simulink model "clutch_trial"  (R2024b)
settings: Solver=ode1be  StartTime=0.0  StopTime=4  FixedStep=0.01  RelTol=1e-3
undefined symbols (not defined in the file or in its folder): J_load, J_rotor, mi_c, mi_s, N_clutch, r_eq_clutch, rpm_in, sigma0, sigma1, sigma2, time, vs
libraries: simulink x3
settings Model: Creator=menda  LastModifiedBy=menda

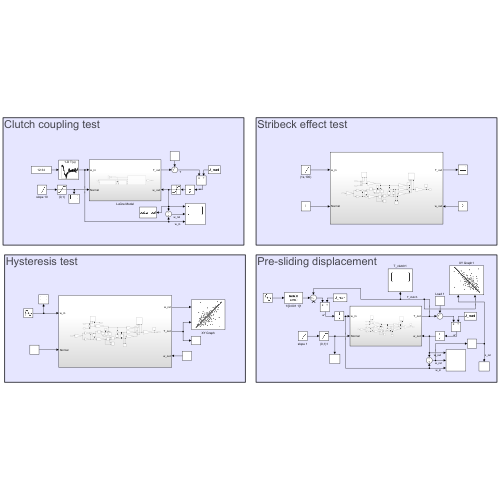
[thumbnail: Simulink's stored preview of the top-level diagram]
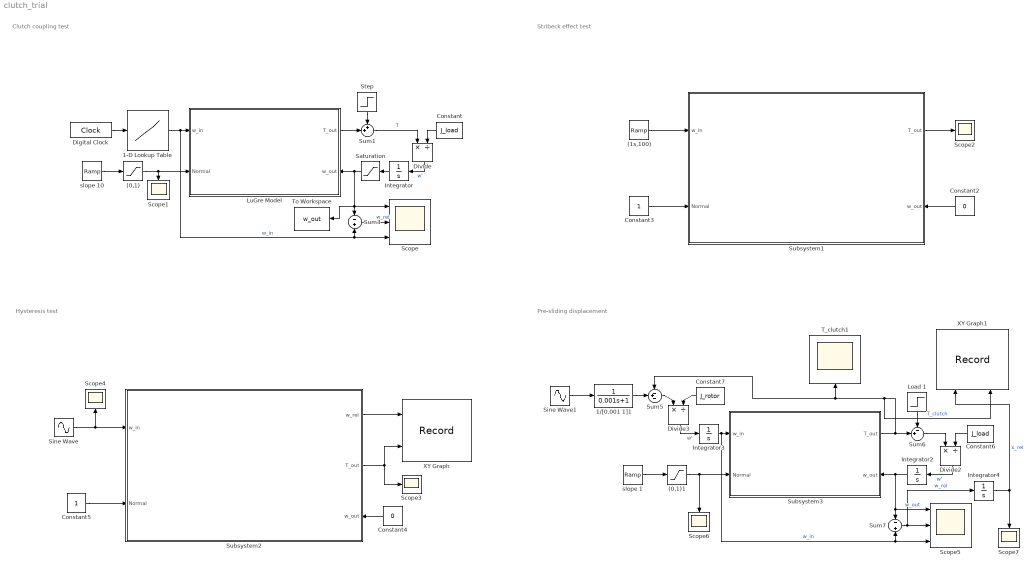
== system clutch_trial ==
  note: Clutch coupling test
  note: Stribeck effect test
  note: Hysteresis test
  note: Pre-sliding displacement
  (0,1) : Saturate  UpperLimit=1  LowerLimit=0
  (0,1)1 : Saturate  UpperLimit=1  LowerLimit=0
  (1s,100) : simulink/Sources/Ramp  slope=100  start=1  InitialOutput=0
  1-D Lookup Table : Lookup_n-D  NumberOfTableDimensions=1  BreakpointsForDimension1=time  Table=rpm_in  InternalRulePriority=Speed  RndMeth=Simplest
  1/[0.001 1]1 : TransferFcn  Denominator=[0.001 1]
  Constant : Constant  Value=J_load
  Constant2 : Constant  Value=0
  Constant3 : Constant
  Constant4 : Constant  Value=0
  Constant5 : Constant
  Constant6 : Constant  Value=J_load
  Constant7 : Constant  Value=J_rotor
  Digital Clock : DigitalClock  SampleTime=0.01
  Divide : Product  Inputs=*/
  Divide2 : Product  Inputs=*/
  Divide3 : Product  Inputs=*/
  Integrator{,2..4} (4 alike) : Integrator
  Load 1 : Step  Time=0  After=0  SampleTime=0
  LuGre Model : Subsystem
      settings: PortSchema="{\"entries\":[{\"content\":{\"sides\":[{\"content\":{\"connectorIds\":[\"In1\",\"In2\"]},\"type\":\"ConnectorPlacement.EquallySpacedRectSide\",\"uuid\":\"4a43e1ea-51cc-4f14-abc2-c6b93b5ec80a\"},{\"content\":{\"connectorIds\":[\"Out1\",\"In3\"],\"side\":\"RIGHT\"},\"type\":\"ConnectorPlacement.EquallySpacedRectSide\",\"uuid\":\"02b73943-aa72-4ec9-9088-698ba8727517\"},{\"content\":{\"side\":\"TOP\"},\"type\":\"ConnectorPlacement.EquallySpacedRectSide\",\"uuid\":\"deeff554-d171-484d-b470-fd1118263e94\"}]},\"type\":\"ConnectorPlacement.EquallySpacedConnector\",\"uuid\":\"dd3f8be3-8b87-48df-afb6-ff993e210eb5\"}],\"packageUris\":[\"http://schema.mathworks.com/mf0/Connector/R2020b\"],\"version\":\"1.0\"}"
  Saturation : Saturate  UpperLimit=inf  LowerLimit=0
  Scope : Scope  NumInputPorts=3
  Scope{1..4,6..7} (6 alike) : Scope
  Scope5 : Scope  NumInputPorts=3
  Sine Wave : Sin  Amplitude=30  Frequency=2  SampleTime=0
  Sine Wave1 : Sin  Amplitude=5  SampleTime=0
  Step : Step  Time=0  After=-10  SampleTime=0
  Subsystem1 : Subsystem
      settings: PortSchema="{\"entries\":[{\"content\":{\"sides\":[{\"content\":{\"connectorIds\":[\"In1\",\"In2\"]},\"type\":\"ConnectorPlacement.EquallySpacedRectSide\",\"uuid\":\"4a43e1ea-51cc-4f14-abc2-c6b93b5ec80a\"},{\"content\":{\"connectorIds\":[\"Out1\",\"In3\"],\"side\":\"RIGHT\"},\"type\":\"ConnectorPlacement.EquallySpacedRectSide\",\"uuid\":\"02b73943-aa72-4ec9-9088-698ba8727517\"},{\"content\":{\"side\":\"TOP\"},\"type\":\"ConnectorPlacement.EquallySpacedRectSide\",\"uuid\":\"deeff554-d171-484d-b470-fd1118263e94\"}]},\"type\":\"ConnectorPlacement.EquallySpacedConnector\",\"uuid\":\"dd3f8be3-8b87-48df-afb6-ff993e210eb5\"}],\"packageUris\":[\"http://schema.mathworks.com/mf0/Connector/R2020b\"],\"version\":\"1.0\"}"
  Subsystem2 : Subsystem
      settings: PortSchema="{\"entries\":[{\"content\":{\"sides\":[{\"content\":{\"connectorIds\":[\"In1\",\"In2\"]},\"type\":\"ConnectorPlacement.EquallySpacedRectSide\",\"uuid\":\"4a43e1ea-51cc-4f14-abc2-c6b93b5ec80a\"},{\"content\":{\"connectorIds\":[\"Out1\",\"Out2\",\"In3\"],\"side\":\"RIGHT\"},\"type\":\"ConnectorPlacement.EquallySpacedRectSide\",\"uuid\":\"02b73943-aa72-4ec9-9088-698ba8727517\"},{\"content\":{\"side\":\"TOP\"},\"type\":\"ConnectorPlacement.EquallySpacedRectSide\",\"uuid\":\"deeff554-d171-484d-b470-fd1118263e94\"}]},\"type\":\"ConnectorPlacement.EquallySpacedConnector\",\"uuid\":\"dd3f8be3-8b87-48df-afb6-ff993e210eb5\"}],\"packageUris\":[\"http://schema.mathworks.com/mf0/Connector/R2020b\"],\"version\":\"1.0\"}"
  Subsystem3 : Subsystem
      settings: PortSchema="{\"entries\":[{\"content\":{\"sides\":[{\"content\":{\"connectorIds\":[\"In1\",\"In2\"]},\"type\":\"ConnectorPlacement.EquallySpacedRectSide\",\"uuid\":\"4a43e1ea-51cc-4f14-abc2-c6b93b5ec80a\"},{\"content\":{\"connectorIds\":[\"Out1\",\"In3\"],\"side\":\"RIGHT\"},\"type\":\"ConnectorPlacement.EquallySpacedRectSide\",\"uuid\":\"02b73943-aa72-4ec9-9088-698ba8727517\"},{\"content\":{\"side\":\"TOP\"},\"type\":\"ConnectorPlacement.EquallySpacedRectSide\",\"uuid\":\"deeff554-d171-484d-b470-fd1118263e94\"}]},\"type\":\"ConnectorPlacement.EquallySpacedConnector\",\"uuid\":\"dd3f8be3-8b87-48df-afb6-ff993e210eb5\"}],\"packageUris\":[\"http://schema.mathworks.com/mf0/Connector/R2020b\"],\"version\":\"1.0\"}"
  Sum1 : Sum  Inputs=++|
  Sum3 : Sum  Inputs=-|+
  Sum5 : Sum  Inputs=-+-
  Sum6 : Sum  Inputs=-+|
  Sum7 : Sum  Inputs=-|+
  T_clutch1 : Scope
  To Workspace : ToWorkspace  VariableName=w_out  SampleTime=-1
  XY Graph : Record  FileSettingsInternal="{\"entries\":[{\"content\":{\"excelSettings\":{\"content\":{},\"type\":\"Streamout.ExcelSettings\"}},\"type\":\"Streamout.FileSettingStorage\",\"uuid\":\"\"}],\"packageUris\":[\"http:\\/\\/schema.mathworks.com\\/mf0\\/streamout_blocks\\/R2020a\"],\"version\":\"1.0\"}"  Layout=[1 1]  SignalsInternal="{\"entries\":[{\"content\":{\"signals\":[{\"content\":{\"blockPath\":[],\"dimensions\":[1],\"domain\":\"\",\"lineColor\":\"#a2142f\",\"plots\":[ 1 ],\"port\":1,\"sid\":[\"\"],\"signalID\":1,\"signalName\":\"Subsystem2:1\"},\"type\":\"RecordBlkView.Signal\",\"uuid\":\"\"},{\"content\":{\"blockPath\":[],\"dimensions\":[1],\"domain\":\"\",\"lineColor\":\"#139fff\",\"plots\":[ 1 ],\"port\":2,\"sid\":[\"\"],\"signalID\":2,\"signalName\":\"Subsystem2:2\"},\"type\":\"RecordBlkView.Signal\",\"uuid\":\"\"}]},\"type\":\"RecordBlkView.InputSignals\",\"uuid\":\"\"}],\"packageUris\":[\"http:\\/\\/schema.mathworks.com\\/mf0\\/streamout_blocks\\/R2020a\"],\"version\":\"1.0\"}"  VisualizationBindings="{\"xyplotplugin\":{\"info\":[{\"series\":[{\"bindingParametersList\":[{\"parameter\":\"X-Axis\",\"signalID\":1,\"signalName\":\"Subsystem2:1\"},{\"parameter\":\"Y-Axis\",\"signalID\":2,\"signalName\":\"Subsystem2:2\"}],\"seriesID\":0}],\"subplotID\":1}]}}"  CompatibilityTag=XY
  XY Graph1 : Record  FileSettingsInternal="{\"entries\":[{\"content\":{\"excelSettings\":{\"content\":{},\"type\":\"Streamout.ExcelSettings\"}},\"type\":\"Streamout.FileSettingStorage\",\"uuid\":\"\"}],\"packageUris\":[\"http:\\/\\/schema.mathworks.com\\/mf0\\/streamout_blocks\\/R2020a\"],\"version\":\"1.0\"}"  Layout=[1 1]  SignalsInternal="{\"entries\":[{\"content\":{\"signals\":[{\"content\":{\"blockPath\":[],\"dimensions\":[1],\"domain\":\"\",\"lineColor\":\"#a2142f\",\"plots\":[ 1 ],\"port\":1,\"sid\":[\"\"],\"signalID\":1,\"signalName\":\"x_rel\"},\"type\":\"RecordBlkView.Signal\",\"uuid\":\"\"},{\"content\":{\"blockPath\":[],\"dimensions\":[1],\"domain\":\"\",\"lineColor\":\"#139fff\",\"plots\":[ 1 ],\"port\":2,\"sid\":[\"\"],\"signalID\":2,\"signalName\":\"T_clutch\"},\"type\":\"RecordBlkView.Signal\",\"uuid\":\"\"}]},\"type\":\"RecordBlkView.InputSignals\",\"uuid\":\"\"}],\"packageUris\":[\"http:\\/\\/schema.mathworks.com\\/mf0\\/streamout_blocks\\/R2020a\"],\"version\":\"1.0\"}"  VisualizationBindings="{\"xyplotplugin\":{\"info\":[{\"series\":[{\"bindingParametersList\":[{\"parameter\":\"X-Axis\",\"signalID\":1,\"signalName\":\"x_rel\"},{\"parameter\":\"Y-Axis\",\"signalID\":2,\"signalName\":\"T_clutch\"}],\"seriesID\":0}],\"subplotID\":1}]}}"  CompatibilityTag=XY
  slope 1 : simulink/Sources/Ramp  slope=10  start=0  InitialOutput=0
  slope 10 : simulink/Sources/Ramp  slope=1  start=0.7  InitialOutput=0
  wires:
  1-D Lookup Table/1 -> Scope/3, Sum3/2, LuGre Model/1(w_in)  "w_in"
  Integrator/1 -> Saturation/1
  Divide/1 -> Integrator/1  "w'"
  slope 10/1 -> (0,1)/1
  (0,1)/1 -> LuGre Model/2(Normal), Scope1/1
  Subsystem1/1(T_out) -> Scope2/1
  Constant2/1 -> Subsystem1/3(w_out)
  Constant3/1 -> Subsystem1/2(Normal)
  (1s,100)/1 -> Subsystem1/1(w_in)
  LuGre Model/1(T_out) -> Sum1/2
  Constant/1 -> Divide/2
  Constant5/1 -> Subsystem2/2(Normal)
  Constant4/1 -> Subsystem2/3(w_out)
  Subsystem2/2(T_out) -> XY Graph/2, Scope3/1
  Sine Wave/1 -> Subsystem2/1(w_in), Scope4/1
  Sum3/1 -> Scope/2  "w_rel"
  Subsystem2/1(w_rel) -> XY Graph/1
  Sum7/1 -> Integrator4/1, Scope5/2  "w_rel"
  Constant6/1 -> Divide2/2
  Sum6/1 -> Divide2/1
  Load 1/1 -> Sum6/1
  1/[0.001 1]1/1 -> Sum5/2
  Sum5/1 -> Divide3/1
  Constant7/1 -> Divide3/2
  Sine Wave1/1 -> 1/[0.001 1]1/1
  (0,1)1/1 -> Scope6/1, Subsystem3/2(Normal)
  Divide3/1 -> Integrator3/1  "w'"
  slope 1/1 -> (0,1)1/1
  Divide2/1 -> Integrator2/1  "w'"
  Subsystem3/1(T_out) -> Sum6/2, T_clutch1/1, Sum5/1, XY Graph1/2  "T_clutch"
  Integrator2/1 -> Scope5/1, Sum7/1, Subsystem3/3(w_out)  "w_out"
  Integrator3/1 -> Subsystem3/1(w_in), Sum7/2, Scope5/3  "w_in"
  Integrator4/1 -> Scope7/1, XY Graph1/1  "x_rel"
  Digital Clock/1 -> 1-D Lookup Table/1
  Sum1/1 -> Divide/1  "T"
  Step/1 -> Sum1/1
  Saturation/1 -> To Workspace/1, Sum3/1, Scope/1, LuGre Model/3(w_out)

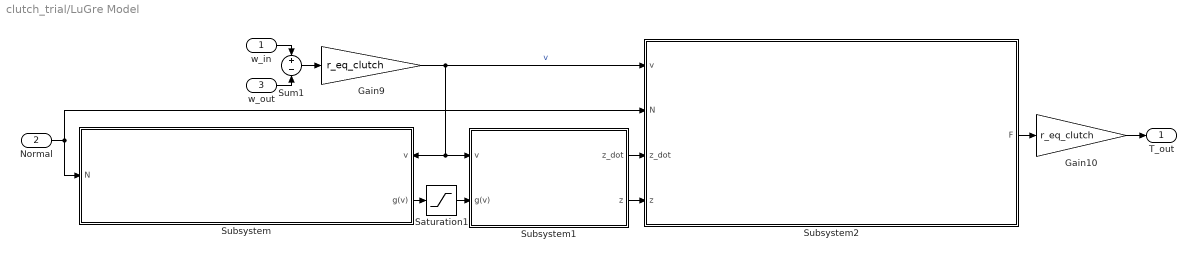
== system clutch_trial/LuGre Model ==
  w_in : Inport
  Normal : Inport  Port=2
  w_out : Inport  Port=3
  Gain10 : Gain  Gain=r_eq_clutch
  Gain9 : Gain  Gain=r_eq_clutch
  Saturation1 : Saturate  UpperLimit=inf  LowerLimit=0.0001
  Subsystem : Subsystem
      settings: PortSchema="{\"entries\":[{\"content\":{\"sides\":[{\"content\":{\"connectorIds\":[\"In1\"]},\"type\":\"ConnectorPlacement.EquallySpacedRectSide\",\"uuid\":\"0ae2ed28-5be6-4ce0-b87c-2c13a72d1ad0\"},{\"content\":{\"connectorIds\":[\"In2\",\"Out1\"],\"side\":\"RIGHT\"},\"type\":\"ConnectorPlacement.EquallySpacedRectSide\",\"uuid\":\"8d48d664-ebaf-4c3e-be9e-f793543e8061\"},{\"content\":{\"side\":\"TOP\"},\"type\":\"ConnectorPlacement.EquallySpacedRectSide\",\"uuid\":\"2d66836a-de46-4974-a48b-ee2778be1c08\"}]},\"type\":\"ConnectorPlacement.EquallySpacedConnector\",\"uuid\":\"ae24f926-3a59-4a74-9cf0-af55dcfbad19\"}],\"packageUris\":[\"http://schema.mathworks.com/mf0/Connector/R2020b\"],\"version\":\"1.0\"}"
      mask Display: image('images/Stribeck.png');
  Subsystem1 : Subsystem
      mask Display: image('images/z_state.png');
  Subsystem2 : Subsystem
      mask Display: image('images/fric_force.png');
  Sum1 : Sum  Inputs=+|-
  T_out : Outport
  wires:
  w_out/1 -> Sum1/2
  w_in/1 -> Sum1/1
  Sum1/1 -> Gain9/1
  Subsystem/1(g(v)) -> Saturation1/1
  Subsystem1/1(z_dot) -> Subsystem2/3(z_dot)
  Gain10/1 -> T_out/1
  Gain9/1 -> Subsystem/2(v), Subsystem1/1(v), Subsystem2/1(v)  "v"
  Subsystem2/1(F) -> Gain10/1
  Subsystem1/2(z) -> Subsystem2/4(z)
  Saturation1/1 -> Subsystem1/2(g(v))
  Normal/1 -> Subsystem/1(N), Subsystem2/2(N)

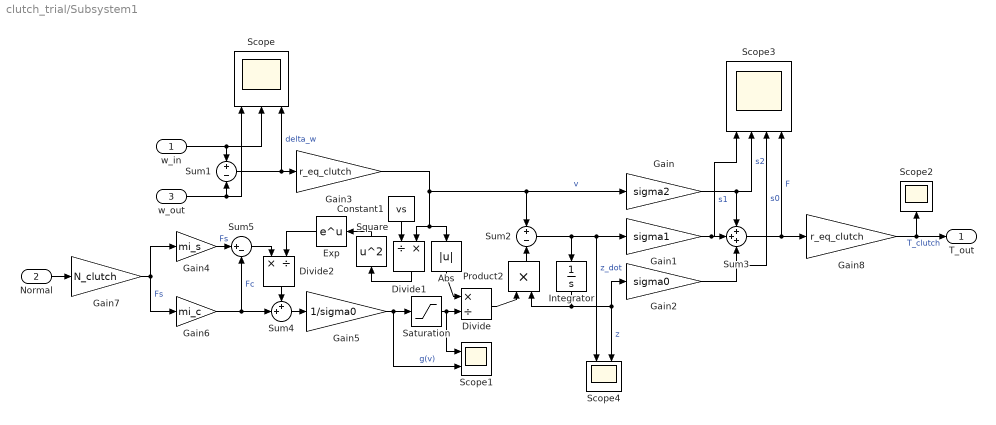
== system clutch_trial/Subsystem1 ==
  w_in : Inport
  Normal : Inport  Port=2
  w_out : Inport  Port=3
  Abs : Abs  SaturateOnIntegerOverflow=off
  Constant1 : Constant  Value=vs
  Divide : Product  Inputs=*/
  Divide1 : Product  Inputs=/*
  Divide2 : Product  Inputs=*/
  Exp : Math
  Gain : Gain  Gain=sigma2
  Gain1 : Gain  Gain=sigma1
  Gain2 : Gain  Gain=sigma0
  Gain3 : Gain  Gain=r_eq_clutch
  Gain4 : Gain  Gain=mi_s
  Gain5 : Gain  Gain=1/sigma0
  Gain6 : Gain  Gain=mi_c
  Gain7 : Gain  Gain=N_clutch
  Gain8 : Gain  Gain=r_eq_clutch
  Integrator : Integrator
  Product2 : Product
  Saturation : Saturate  UpperLimit=inf  LowerLimit=0.0001
  Scope : Scope  NumInputPorts=3
  Scope1 : Scope  NumInputPorts=2
  Scope2 : Scope
  Scope3 : Scope  NumInputPorts=4
  Scope4 : Scope  NumInputPorts=2
  Square : Math  Operator=square
  Sum1 : Sum  Inputs=+|-
  Sum2 : Sum  Inputs=+|-
  Sum3 : Sum  Inputs=+++
  Sum4 : Sum  Inputs=++|
  Sum5 : Sum  Inputs=|+-
  T_out : Outport
  wires:
  Gain1/1 -> Scope3/1, Sum3/2  "s1"
  Gain5/1 -> Saturation/1, Scope1/2  "g(v)"
  Gain2/1 -> Scope3/3, Sum3/3  "s0"
  w_out/1 -> Scope/1, Sum1/2
  Gain4/1 -> Sum5/1  "Fs"
  Sum1/1 -> Gain3/1, Scope/3  "delta_w"
  Gain7/1 -> Gain6/1, Gain4/1  "Fs"
  Normal/1 -> Gain7/1
  Exp/1 -> Divide2/2
  Gain8/1 -> T_out/1, Scope2/1  "T_clutch"
  Divide1/1 -> Square/1
  Divide/1 -> Product2/1
  Product2/1 -> Sum2/2
  Sum3/1 -> Gain8/1, Scope3/4  "F"
  Gain6/1 -> Sum4/2, Sum5/2  "Fc"
  Abs/1 -> Divide/1
  Constant1/1 -> Divide1/1
  Gain3/1 -> Sum2/1, Gain/1, Abs/1, Divide1/2  "v"
  Sum2/1 -> Gain1/1, Scope4/1, Integrator/1  "z_dot"
  Divide2/1 -> Sum4/1
  Square/1 -> Exp/1
  Sum4/1 -> Gain5/1
  Gain/1 -> Scope3/2, Sum3/1  "s2"
  w_in/1 -> Scope/2, Sum1/1
  Integrator/1 -> Scope4/2, Gain2/1, Product2/2  "z"
  Sum5/1 -> Divide2/1
  Saturation/1 -> Scope1/1, Divide/2

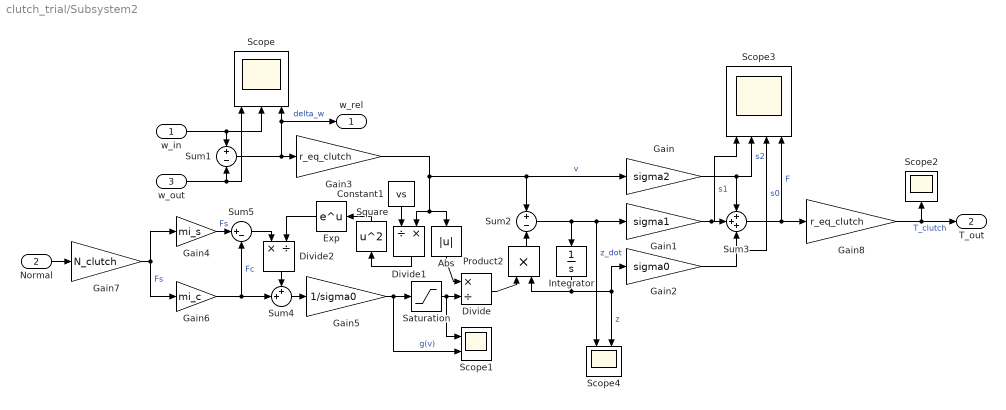
== system clutch_trial/Subsystem2 ==
  w_in : Inport
  Normal : Inport  Port=2
  w_out : Inport  Port=3
  Abs : Abs  SaturateOnIntegerOverflow=off
  Constant1 : Constant  Value=vs
  Divide : Product  Inputs=*/
  Divide1 : Product  Inputs=/*
  Divide2 : Product  Inputs=*/
  Exp : Math
  Gain : Gain  Gain=sigma2
  Gain1 : Gain  Gain=sigma1
  Gain2 : Gain  Gain=sigma0
  Gain3 : Gain  Gain=r_eq_clutch
  Gain4 : Gain  Gain=mi_s
  Gain5 : Gain  Gain=1/sigma0
  Gain6 : Gain  Gain=mi_c
  Gain7 : Gain  Gain=N_clutch
  Gain8 : Gain  Gain=r_eq_clutch
  Integrator : Integrator
  Product2 : Product
  Saturation : Saturate  UpperLimit=inf  LowerLimit=0.0001
  Scope : Scope  NumInputPorts=3
  Scope1 : Scope  NumInputPorts=2
  Scope2 : Scope
  Scope3 : Scope  NumInputPorts=4
  Scope4 : Scope  NumInputPorts=2
  Square : Math  Operator=square
  Sum1 : Sum  Inputs=+|-
  Sum2 : Sum  Inputs=+|-
  Sum3 : Sum  Inputs=+++
  Sum4 : Sum  Inputs=++|
  Sum5 : Sum  Inputs=|+-
  w_rel : Outport
  T_out : Outport  Port=2
  wires:
  Saturation/1 -> Divide/2, Scope1/1
  Sum5/1 -> Divide2/1
  Integrator/1 -> Product2/2, Gain2/1, Scope4/2  "z"
  w_in/1 -> Sum1/1, Scope/2
  Gain/1 -> Sum3/1, Scope3/2  "s2"
  Sum4/1 -> Gain5/1
  Square/1 -> Exp/1
  Divide2/1 -> Sum4/1
  Sum2/1 -> Integrator/1, Scope4/1, Gain1/1  "z_dot"
  Gain3/1 -> Divide1/2, Abs/1, Gain/1, Sum2/1  "v"
  Constant1/1 -> Divide1/1
  Abs/1 -> Divide/1
  Gain6/1 -> Sum5/2, Sum4/2  "Fc"
  Sum3/1 -> Scope3/4, Gain8/1  "F"
  Product2/1 -> Sum2/2
  Divide/1 -> Product2/1
  Divide1/1 -> Square/1
  Gain8/1 -> T_out/1, Scope2/1  "T_clutch"
  Exp/1 -> Divide2/2
  Normal/1 -> Gain7/1
  Gain7/1 -> Gain4/1, Gain6/1  "Fs"
  Sum1/1 -> w_rel/1, Scope/3, Gain3/1  "delta_w"
  Gain4/1 -> Sum5/1  "Fs"
  w_out/1 -> Sum1/2, Scope/1
  Gain2/1 -> Sum3/3, Scope3/3  "s0"
  Gain5/1 -> Scope1/2, Saturation/1  "g(v)"
  Gain1/1 -> Sum3/2, Scope3/1  "s1"

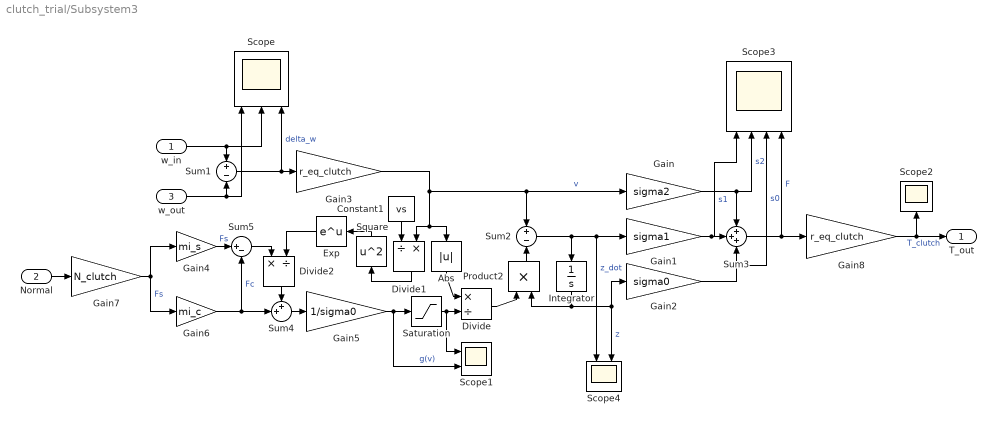
== system clutch_trial/Subsystem3 ==
  w_in : Inport
  Normal : Inport  Port=2
  w_out : Inport  Port=3
  Abs : Abs  SaturateOnIntegerOverflow=off
  Constant1 : Constant  Value=vs
  Divide : Product  Inputs=*/
  Divide1 : Product  Inputs=/*
  Divide2 : Product  Inputs=*/
  Exp : Math
  Gain : Gain  Gain=sigma2
  Gain1 : Gain  Gain=sigma1
  Gain2 : Gain  Gain=sigma0
  Gain3 : Gain  Gain=r_eq_clutch
  Gain4 : Gain  Gain=mi_s
  Gain5 : Gain  Gain=1/sigma0
  Gain6 : Gain  Gain=mi_c
  Gain7 : Gain  Gain=N_clutch
  Gain8 : Gain  Gain=r_eq_clutch
  Integrator : Integrator
  Product2 : Product
  Saturation : Saturate  UpperLimit=inf  LowerLimit=0.0001
  Scope : Scope  NumInputPorts=3
  Scope1 : Scope  NumInputPorts=2
  Scope2 : Scope
  Scope3 : Scope  NumInputPorts=4
  Scope4 : Scope  NumInputPorts=2
  Square : Math  Operator=square
  Sum1 : Sum  Inputs=+|-
  Sum2 : Sum  Inputs=+|-
  Sum3 : Sum  Inputs=+++
  Sum4 : Sum  Inputs=++|
  Sum5 : Sum  Inputs=|+-
  T_out : Outport
  wires:
  Saturation/1 -> Divide/2, Scope1/1
  Sum5/1 -> Divide2/1
  Integrator/1 -> Product2/2, Gain2/1, Scope4/2  "z"
  w_in/1 -> Sum1/1, Scope/2
  Gain/1 -> Sum3/1, Scope3/2  "s2"
  Sum4/1 -> Gain5/1
  Square/1 -> Exp/1
  Divide2/1 -> Sum4/1
  Sum2/1 -> Integrator/1, Scope4/1, Gain1/1  "z_dot"
  Gain3/1 -> Divide1/2, Abs/1, Gain/1, Sum2/1  "v"
  Constant1/1 -> Divide1/1
  Abs/1 -> Divide/1
  Gain6/1 -> Sum5/2, Sum4/2  "Fc"
  Sum3/1 -> Scope3/4, Gain8/1  "F"
  Product2/1 -> Sum2/2
  Divide/1 -> Product2/1
  Divide1/1 -> Square/1
  Gain8/1 -> Scope2/1, T_out/1  "T_clutch"
  Exp/1 -> Divide2/2
  Normal/1 -> Gain7/1
  Gain7/1 -> Gain4/1, Gain6/1  "Fs"
  Sum1/1 -> Scope/3, Gain3/1  "delta_w"
  Gain4/1 -> Sum5/1  "Fs"
  w_out/1 -> Sum1/2, Scope/1
  Gain2/1 -> Sum3/3, Scope3/3  "s0"
  Gain5/1 -> Scope1/2, Saturation/1  "g(v)"
  Gain1/1 -> Sum3/2, Scope3/1  "s1"

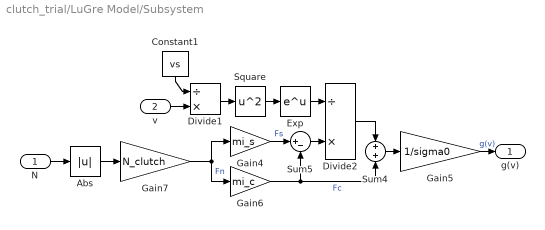
== system clutch_trial/LuGre Model/Subsystem ==
  N : Inport
  v : Inport  Port=2
  Abs : Abs  SaturateOnIntegerOverflow=off
  Constant1 : Constant  Value=vs
  Divide1 : Product  Inputs=/*
  Divide2 : Product  Inputs=/*
  Exp : Math
  Gain4 : Gain  Gain=mi_s
  Gain5 : Gain  Gain=1/sigma0
  Gain6 : Gain  Gain=mi_c
  Gain7 : Gain  Gain=N_clutch
  Square : Math  Operator=square
  Sum4 : Sum  Inputs=+|+
  Sum5 : Sum  Inputs=|+-
  g(v) : Outport
  wires:
  Gain4/1 -> Sum5/1  "Fs"
  Abs/1 -> Gain7/1
  v/1 -> Divide1/2
  N/1 -> Abs/1
  Gain5/1 -> g(v)/1  "g(v)"
  Square/1 -> Exp/1
  Divide1/1 -> Square/1
  Constant1/1 -> Divide1/1
  Gain7/1 -> Gain4/1, Gain6/1  "Fn"
  Exp/1 -> Divide2/1
  Gain6/1 -> Sum5/2, Sum4/2  "Fc"
  Divide2/1 -> Sum4/1
  Sum5/1 -> Divide2/2
  Sum4/1 -> Gain5/1

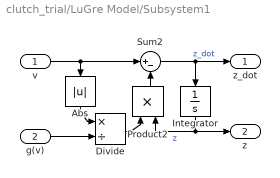
== system clutch_trial/LuGre Model/Subsystem1 ==
  v : Inport
  g(v) : Inport  Port=2
  Abs : Abs  SaturateOnIntegerOverflow=off
  Divide : Product  Inputs=*/
  Integrator : Integrator
  Product2 : Product
  Sum2 : Sum  Inputs=|+-
  z_dot : Outport
  z : Outport  Port=2
  wires:
  g(v)/1 -> Divide/2
  v/1 -> Abs/1, Sum2/1
  Integrator/1 -> Product2/2, z/1  "z"
  Sum2/1 -> Integrator/1, z_dot/1  "z_dot"
  Divide/1 -> Product2/1
  Abs/1 -> Divide/1
  Product2/1 -> Sum2/2

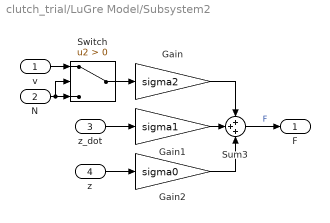
== system clutch_trial/LuGre Model/Subsystem2 ==
  v : Inport
  N : Inport  Port=2
  z_dot : Inport  Port=3
  z : Inport  Port=4
  Gain : Gain  Gain=sigma2
  Gain1 : Gain  Gain=sigma1
  Gain2 : Gain  Gain=sigma0
  Sum3 : Sum  Inputs=+++
  Switch : Switch  Criteria=u2 > Threshold  SaturateOnIntegerOverflow=off  InputSameDT=off
  F : Outport
  wires:
  z/1 -> Gain2/1
  v/1 -> Switch/1
  z_dot/1 -> Gain1/1
  Gain1/1 -> Sum3/2
  Sum3/1 -> F/1  "F"
  Gain2/1 -> Sum3/3
  Gain/1 -> Sum3/1
  N/1 -> Switch/2, Switch/3
  Switch/1 -> Gain/1
